simulink model "part2_MAIN_2019_for_ayon_because_he_cant_update_his_matlab"  (R2019a)
settings: Solver=FixedStepAuto  StartTime=0.0  StopTime=300  FixedStep=0.1  RelTol=1e-3
values from neighbouring files (symbols this model uses):
  Af = diag(ti)    [init.m]    (also in init_old.m)
  Aw = [zeros(3) eye(3) ... (first row only)    [get_observer_parameters.m]
  B = [thr1 thr2_x thr2_y thr3 thr4_x thr4_y thr5_x thr5_y]    [B_redistributed.m]    (also in check_alg.m = [1 2 3 4 5 6 7 8; get_observer_parameters.m = [zeros(6,3);zeros(3,3);zeros(3,3);inv(M)])
  change_position_time = 1200    [init.m]    (also in init_old.m)
  Cw = [zeros(3) eye(3)]    [get_observer_parameters.m]
  D = Damping    [init.m]    (also in init_old.m)
  Damping = diag([2.6486e5, 8.8164e5, 3.3774e8])    [init.m]    (also in init_old.m)
  direction_limit = pi/36    (= 0.0872664625997)    [init.m]    (also in init_old.m)
  direction_time_constant = 100    [init.m]    (also in init_old.m)
  dt = 0.1    [get_observer_parameters.m]
  E = [Ew, zeros(6,3) ... (first row only)    [get_observer_parameters.m]
  Gamma = diag(omega_is)    [init.m]    (also in init_old.m)
  gust_limit = 40    [init.m]    (also in init_old.m)
  H = [Cw, eye(3), zeros(3,3) zeros(3,3)]    [get_observer_parameters.m]    (also in quadprog.m = 2*diag([w.' w.' q.' q.' w_alpha.' w_alpha.']); quadprog_basic.m = 2*diag([w.' w.' q.' q.']); quadprog_false.m = 2*diag([w.' w.' q.' q.' w_alpha.' w_alpha.']))
  height = 3    [init.m]    (also in init_old.m)
  inv_M = inv(M)    [get_observer_parameters.m]
  inv_Tb = inv(Tb)    [get_observer_parameters.m]
  kappa = 0.003    [init.m]    (also in init_old.m)
  kappa2 = 0.0026    [init.m]    (also in init_old.m)
  Kd = [1660451.40544401; 3920391.80535684; 1605063439.04156]    [init.m]    (also in init_old.m)
  Ki = [137.081306245593; 3163.274947400198; 335358.448218978]    [init.m]    (also in init_old.m)
  Kp = [75459.3345349083; 277551.73586971; 120744473.878042]    [init.m]    (also in init_old.m)
  L = 1800    [init.m]    (also in init_old.m)
  M = Mass    [init.m]    (also in init_old.m)
  mean_wind_direction = pi    (= 3.14159265359)    [init.m]    (also in init_old.m)
  observer_type = 0    [init.m]    (also in init_old.m)
  Omega = diag([omega_n, omega_n, omega_n])    [get_observer_parameters.m]    (also in init.m = diag(2*omega_is.*zeta_is); init_old.m = diag(2*omega_is.*zeta_is))
  Q = diag([0.1,0.1,pi/180,1e6,1e6,1e9])*10e3    [get_observer_parameters.m]
  R = diag([1,0.1,0.1*pi/180])*10e-3    [get_observer_parameters.m]
  simulation = 7    [init.m]    (also in init_old.m = 1)
  slow_varying_limit = 1    [init.m]    (also in init_old.m)
  slow_varying_time_constant = 100    [init.m]    (also in init_old.m)
  TAU = dt*E    [get_observer_parameters.m]
  Tb = 0.1 * eye(3)    [get_observer_parameters.m]
  thruster_type = 0    [init.m]    (also in init_old.m)
  u10 = 12    [init.m]    (also in init_old.m)
  vessel =     [test.mat]
  wind = 1    [init.m]    (also in init_old.m)
undefined symbols (not defined in the file or in its folder): Hoerner, ModelParams, npf, Param, thrusters, WaveModel
libraries: simulink x49, dspsigops x39, marine_hydro x14, marine_gnc x7
(part 5 of 9)

== system part2_MAIN_2019_for_ayon_because_he_cant_update_his_matlab/ Original/Wind/V_w1 ==
  " " : Constant  Value=mean_wind_direction
  Band-Limited White Noise : simulink/Sources/Band-Limited White Noise  Cov=np_slow_varying  Ts=0.1  seed=[23341]
  Band-Limited White Noise1 : simulink/Sources/Band-Limited White Noise  Cov=np_direction  Ts=0.1  seed=[23341]
  Constant : Constant  Value=u10
  Constant1 : Constant  Value=kappa
  Constant2 : Constant  Value=height
  Constant3 : Constant  Value=u10
  Constant8 : Constant  Value=L
  Constant9 : Constant  Value=kappa2
  Gain : Gain  Gain=1/slow_varying_time_constant
  Gain1 : Gain  Gain=1/direction_time_constant
  Gust : MATLAB Function  TreatAsAtomicUnit=on
  Integrator : Integrator  LimitOutput=on  UpperSaturationLimit=slow_varying_limit  LowerSaturationLimit=-slow_varying_limit
  Integrator1 : Integrator  LimitOutput=on  UpperSaturationLimit=direction_limit  LowerSaturationLimit=-direction_limit
  Mean wind component : MATLAB Function  TreatAsAtomicUnit=on
  Saturation : Saturate  UpperLimit=gust_limit  LowerLimit=-10
  Scope{,1..3} (4 alike) : Scope
  Sum : Sum  Inputs=+|+|+
  Sum1 : Sum  Inputs=|+-
  Sum2 : Sum  Inputs=|+-
  Sum3 : Sum  Inputs=|++
  time : Clock
  wind : Outport
  direction : Outport  Port=2
  wires:
  Constant3/1 -> Mean wind component/1(u10)
  Constant1/1 -> Mean wind component/2(kappa)
  Constant2/1 -> Mean wind component/3(height)
  Mean wind component/1(mean_wind) -> Scope2/1, Sum/2
  Sum/1 -> wind/1
  Integrator/1 -> Scope1/1, Sum/1, Sum1/2
  Band-Limited White Noise/1 -> Sum1/1
  Integrator1/1 -> Sum2/2, Sum3/1
  Band-Limited White Noise1/1 -> Sum2/1
  " "/1 -> Sum3/2
  Sum3/1 -> Scope3/1, direction/1
  Gain1/1 -> Integrator1/1
  Sum2/1 -> Gain1/1
  Gain/1 -> Integrator/1
  Sum1/1 -> Gain/1
  Constant8/1 -> Gust/3(L)
  Gust/1(gust) -> Saturation/1
  Saturation/1 -> Sum/3, Scope/1
  Constant9/1 -> Gust/4(kappa2)
  Constant/1 -> Gust/2(u10)
  time/1 -> Gust/1(time)

== system part2_MAIN_2019_for_ayon_because_he_cant_update_his_matlab/Simulation 1/Current (North - East)/Subsystem ==
  Mux1 : Mux  Inputs=3
  Scope : Scope
  Step1 : Step  Time=0  After=0  SampleTime=0
  Step2 : Step  Time=0  After=-0.2  SampleTime=0
  Step3 : Step  Time=0  After=0  SampleTime=0
  Out1 : Outport
  wires:
  Mux1/1 -> Scope/1, Out1/1
  Step1/1 -> Mux1/1
  Step2/1 -> Mux1/2
  Step3/1 -> Mux1/3

== system part2_MAIN_2019_for_ayon_because_he_cant_update_his_matlab/Simulation 1/Current (North - East)/Subsystem1 ==
  Add : Sum  Inputs=+++
  Cos : Trigonometry  Operator=cos
  Gain : Gain  Gain=pi/180
  Matrix Multiply : Product
  Matrix Multiply1 : Product
  Mux : Mux  Inputs=3
  Ramp : simulink/Sources/Ramp  slope=0.45  start=2  InitialOutput=0
  Ramp1 : simulink/Sources/Ramp  slope=-0.45  start=202  InitialOutput=0
  Scope : Scope  NumInputPorts=3
  Sin : Trigonometry
  Step : Step  Time=2  After=0.5  SampleTime=0
  Step1 : Step  Time=2  Before=180  After=180  SampleTime=0
  Step2 : Step  Time=0  After=0  SampleTime=0
  Out1 : Outport
  wires:
  Step1/1 -> Add/1
  Ramp/1 -> Add/2
  Ramp1/1 -> Add/3
  Step/1 -> Matrix Multiply1/1, Matrix Multiply/1
  Sin/1 -> Matrix Multiply1/2, Scope/1
  Cos/1 -> Matrix Multiply/2, Scope/2
  Matrix Multiply/1 -> Mux/1
  Matrix Multiply1/1 -> Mux/2
  Step2/1 -> Mux/3
  Mux/1 -> Scope/3, Out1/1
  Add/1 -> Gain/1
  Gain/1 -> Sin/1, Cos/1

== system part2_MAIN_2019_for_ayon_because_he_cant_update_his_matlab/Simulation 1/Current (North - East)/Subsystem2 ==
  Mux : Mux  Inputs=3
  Step : Step  Time=0  After=0  SampleTime=0
  Out1 : Outport
  wires:
  Mux/1 -> Out1/1
  Step/1 -> Mux/3, Mux/2, Mux/1

== system part2_MAIN_2019_for_ayon_because_he_cant_update_his_matlab/Simulation 1/Observer/EKF ==
  note: selector
  y : Inport
  U : Inport  Port=2
  Constant : Constant  Value=M
  Constant1 : Constant  Value=D
  Constant10 : Constant  Value=Q
  Constant11 : Constant  Value=dt
  Constant12 : Constant  Value=inv_Tb
  Constant13 : Constant  Value=TAU
  Constant2 : Constant  Value=inv_M
  Constant3 : Constant  Value=Tb
  Constant4 : Constant  Value=Aw
  Constant5 : Constant  Value=Cw
  Constant6 : Constant  Value=B
  Constant7 : Constant  Value=H
  Constant8 : Constant  Value=E
  Constant9 : Constant  Value=R
  MATLAB Function : MATLAB Function  TreatAsAtomicUnit=on
  MATLAB Function1 : MATLAB Function  TreatAsAtomicUnit=on
  Memory : Memory  InitialCondition=zeros(15,1)
  Memory1 : Memory  InitialCondition=eye(15,15)
  Scope : Scope
  Scope2 : Scope
  Subsystem : Subsystem  Commented=on
  Subsystem1 : Subsystem  Commented=on
  Terminator : Terminator
  eta_hat : Outport
  nu_hat : Outport  Port=2
  wires:
  U/1 -> MATLAB Function/2(U)
  MATLAB Function1/1(eta_hat) -> eta_hat/1
  MATLAB Function/3(states_hat) -> MATLAB Function1/1(states_vector)
  MATLAB Function/4(error) -> Scope2/1
  y/1 -> MATLAB Function/1(y)
  MATLAB Function1/2(nu_hat) -> nu_hat/1
  MATLAB Function/2(states_update) -> Memory/1
  Constant/1 -> MATLAB Function/5(M)
  Constant1/1 -> MATLAB Function/6(D)
  Constant2/1 -> MATLAB Function/7(inv_M)
  Constant4/1 -> MATLAB Function/8(Aw)
  Constant3/1 -> MATLAB Function/9(Tb)
  Constant5/1 -> MATLAB Function/10(Cw)
  Constant8/1 -> MATLAB Function/11(E)
  Constant6/1 -> MATLAB Function/12(B)
  Constant7/1 -> MATLAB Function/13(H)
  Constant9/1 -> MATLAB Function/14(R)
  Constant10/1 -> MATLAB Function/15(Q)
  Constant11/1 -> MATLAB Function/16(dt)
  Constant12/1 -> MATLAB Function/17(inv_Tb)
  Constant13/1 -> MATLAB Function/18(TAU)
  Memory/1 -> MATLAB Function/4(states)
  MATLAB Function/1(P_update) -> Memory1/1, Scope/1
  Memory1/1 -> MATLAB Function/3(P)
  MATLAB Function/5(K) -> Terminator/1

== system part2_MAIN_2019_for_ayon_because_he_cant_update_his_matlab/Simulation 1/Observer/Passive Non-Linear ==
  note: eta_observer
  note: nu_observer
  note: Bias Estimator
  note: Wave Estimator: 1st order wave-induced motion
  y : Inport
  tau_est : Inport  Port=2
  Add : Sum
  Add1 : Sum  Inputs=++-
  Aw : Gain  Gain=WaveModel.A_w  Multiplication=Matrix(K*u)
  Cw : Gain  Gain=WaveModel.C_w  Multiplication=Matrix(K*u)
  Damping : Gain  Gain=Damping  Multiplication=Matrix(K*u)
  Integrator{,1..3} (4 alike) : Integrator
  K1 : Gain  Gain=npf.K_1  Multiplication=Matrix(K*u)
  K2 : Gain  Gain=npf.K_2  Multiplication=Matrix(K*u)
  K3 : Gain  Gain=npf.K_3  Multiplication=Matrix(K*u)
  K4 : Gain  Gain=npf.K_4  Multiplication=Matrix(K*u)
  M_inv : Gain  Gain=inv(ModelParams.Mass)  Multiplication=Matrix(K*u)
  Matrix Multiply : Product  Multiplication=Matrix(*)
  Matrix Multiply1 : Product  Multiplication=Matrix(*)
  Matrix Multiply2 : Product  Multiplication=Matrix(*)
  R_psi : MATLAB Function  TreatAsAtomicUnit=on
  R_psi_T : MATLAB Function  TreatAsAtomicUnit=on
  Subsystem : Subsystem
  Sum : Sum  Inputs=|++
  Sum1 : Sum  Inputs=|+-
  Sum2 : Sum  Inputs=|++
  Sum3 : Sum  Inputs=|++
  Sum4 : Sum  Inputs=|+-
  inv(Tb) : Gain  Gain=inv(Param.Tb)  Multiplication=Matrix(K*u)
  eta_hat : Outport
  nu_hat : Outport  Port=2
  wires:
  Matrix Multiply/1 -> Sum/1
  Matrix Multiply1/1 -> Add/2
  Matrix Multiply2/1 -> Add1/1  "R'b_hat"
  R_psi_T/1(y) -> Matrix Multiply/1, Matrix Multiply2/2
  Add1/1 -> M_inv/1
  Damping/1 -> Add1/3
  R_psi/1(y) -> Matrix Multiply1/1
  Sum/1 -> Add1/2  "R'k4y + tau"
  Add/1 -> Integrator3/1  "eta_hat_dot"
  inv(Tb)/1 -> Sum1/2
  y/1 -> Subsystem/1(y), Sum4/1  "y"
  Aw/1 -> Sum2/2
  K3/1 -> Sum1/1
  Cw/1 -> Sum3/1
  Integrator1/1 -> Cw/1, Aw/1  "zeta_hat"
  Sum1/1 -> Integrator2/1  "b_hat_dot"
  Integrator/1 -> nu_hat/1, Damping/1, Matrix Multiply1/2  "nu_hat"
  Sum4/1 -> K1/1, K2/1, K3/1, K4/1  "y_obs"
  Sum3/1 -> Sum4/2  "y_hat"
  Integrator3/1 -> eta_hat/1, Sum3/2  "eta_hat"
  Sum2/1 -> Integrator1/1
  K2/1 -> Add/1
  K4/1 -> Matrix Multiply/2
  M_inv/1 -> Integrator/1  "nu_hat_dot"
  Integrator2/1 -> inv(Tb)/1, Matrix Multiply2/1  "b_hat"
  tau_est/1 -> Sum/2
  K1/1 -> Sum2/1
  Subsystem/1(Out1) -> R_psi/1(u), R_psi_T/1(u)

== system part2_MAIN_2019_for_ayon_because_he_cant_update_his_matlab/Simulation 1/Observer/Subsystem ==
  In1 : Inport
  Demux : Demux  Outputs=6
  Mux : Mux  Inputs=3
  Terminator : Terminator
  Terminator1 : Terminator
  Terminator2 : Terminator
  Out1 : Outport
  wires:
  Mux/1 -> Out1/1
  Demux/6 -> Mux/3
  Demux/5 -> Terminator2/1
  Demux/2 -> Mux/2
  Demux/1 -> Mux/1
  Demux/3 -> Terminator/1
  In1/1 -> Demux/1
  Demux/4 -> Terminator1/1

== system part2_MAIN_2019_for_ayon_because_he_cant_update_his_matlab/Simulation 1/Reference Model/Simulation Selector ==
  Simulation 4 : Subsystem
  Out1 : Outport
  wires:
  Simulation 4/1(Out1) -> Out1/1

== system part2_MAIN_2019_for_ayon_because_he_cant_update_his_matlab/Simulation 1/Thrust Allocation/Unwrap ==
  alpha : Inport
  Demux : Demux  Outputs=5
  Mux : Mux  Inputs=5
  Unwrap : dspsigops/Unwrap  tol=pi  InputProcessing=Columns as channels (frame based)  running=off
  Unwrap1 : dspsigops/Unwrap  tol=pi  InputProcessing=Columns as channels (frame based)  running=off
  Unwrap2 : dspsigops/Unwrap  tol=pi  InputProcessing=Columns as channels (frame based)  running=off
  alpha [rad] : Outport
  wires:
  alpha/1 -> Demux/1
  Mux/1 -> alpha [rad]/1
  Demux/1 -> Mux/1
  Demux/4 -> Unwrap2/1
  Unwrap2/1 -> Mux/4
  Demux/5 -> Unwrap/1
  Unwrap/1 -> Mux/5
  Demux/3 -> Mux/3
  Demux/2 -> Unwrap1/1
  Unwrap1/1 -> Mux/2

== system part2_MAIN_2019_for_ayon_because_he_cant_update_his_matlab/Simulation 1/Thrust Allocation/Unwrap1 ==
  alpha : Inport
  Demux : Demux  Outputs=5
  Mux : Mux  Inputs=5
  Unwrap : dspsigops/Unwrap  tol=pi  InputProcessing=Columns as channels (frame based)  running=off
  Unwrap1 : dspsigops/Unwrap  tol=pi  InputProcessing=Columns as channels (frame based)  running=off
  Unwrap2 : dspsigops/Unwrap  tol=pi  InputProcessing=Columns as channels (frame based)  running=off
  alpha [rad] : Outport
  wires:
  Unwrap1/1 -> Mux/2
  Demux/2 -> Unwrap1/1
  Demux/3 -> Mux/3
  Unwrap/1 -> Mux/5
  Demux/5 -> Unwrap/1
  Unwrap2/1 -> Mux/4
  Demux/4 -> Unwrap2/1
  Demux/1 -> Mux/1
  Mux/1 -> alpha [rad]/1
  alpha/1 -> Demux/1

== system part2_MAIN_2019_for_ayon_because_he_cant_update_his_matlab/Simulation 1/Wind/V_w1 ==
  " " : Constant  Value=mean_wind_direction
  Band-Limited White Noise : simulink/Sources/Band-Limited White Noise  Cov=np_slow_varying  Ts=0.1  seed=[23341]
  Band-Limited White Noise1 : simulink/Sources/Band-Limited White Noise  Cov=np_direction  Ts=0.1  seed=[23341]
  Constant : Constant  Value=u10
  Constant1 : Constant  Value=kappa
  Constant2 : Constant  Value=height
  Constant3 : Constant  Value=u10
  Constant8 : Constant  Value=L
  Constant9 : Constant  Value=kappa2
  Gain : Gain  Gain=1/slow_varying_time_constant
  Gain1 : Gain  Gain=1/direction_time_constant
  Gust : MATLAB Function  TreatAsAtomicUnit=on
  Integrator : Integrator  LimitOutput=on  UpperSaturationLimit=slow_varying_limit  LowerSaturationLimit=-slow_varying_limit
  Integrator1 : Integrator  LimitOutput=on  UpperSaturationLimit=direction_limit  LowerSaturationLimit=-direction_limit
  Mean wind component : MATLAB Function  TreatAsAtomicUnit=on
  Saturation : Saturate  UpperLimit=gust_limit  LowerLimit=-10
  Scope{,1..3} (4 alike) : Scope
  Sum : Sum  Inputs=+|+|+
  Sum1 : Sum  Inputs=|+-
  Sum2 : Sum  Inputs=|+-
  Sum3 : Sum  Inputs=|++
  time : Clock
  wind : Outport
  direction : Outport  Port=2
  wires:
  Constant3/1 -> Mean wind component/1(u10)
  Constant1/1 -> Mean wind component/2(kappa)
  Constant2/1 -> Mean wind component/3(height)
  Mean wind component/1(mean_wind) -> Scope2/1, Sum/2
  Sum/1 -> wind/1
  Integrator/1 -> Scope1/1, Sum/1, Sum1/2
  Band-Limited White Noise/1 -> Sum1/1
  Integrator1/1 -> Sum2/2, Sum3/1
  Band-Limited White Noise1/1 -> Sum2/1
  " "/1 -> Sum3/2
  Sum3/1 -> Scope3/1, direction/1
  Gain1/1 -> Integrator1/1
  Sum2/1 -> Gain1/1
  Gain/1 -> Integrator/1
  Sum1/1 -> Gain/1
  Constant8/1 -> Gust/3(L)
  Gust/1(gust) -> Saturation/1
  Saturation/1 -> Sum/3, Scope/1
  Constant9/1 -> Gust/4(kappa2)
  Constant/1 -> Gust/2(u10)
  time/1 -> Gust/1(time)

== system part2_MAIN_2019_for_ayon_because_he_cant_update_his_matlab/Simulation 2/Current (North - East)/Subsystem ==
  Mux1 : Mux  Inputs=3
  Scope : Scope
  Step1 : Step  Time=0  After=0  SampleTime=0
  Step2 : Step  Time=0  After=-0.2  SampleTime=0
  Step3 : Step  Time=0  After=0  SampleTime=0
  Out1 : Outport
  wires:
  Mux1/1 -> Scope/1, Out1/1
  Step1/1 -> Mux1/1
  Step2/1 -> Mux1/2
  Step3/1 -> Mux1/3

== system part2_MAIN_2019_for_ayon_because_he_cant_update_his_matlab/Simulation 2/Current (North - East)/Subsystem1 ==
  Add : Sum  Inputs=+++
  Cos : Trigonometry  Operator=cos
  Gain : Gain  Gain=pi/180
  Matrix Multiply : Product
  Matrix Multiply1 : Product
  Mux : Mux  Inputs=3
  Ramp : simulink/Sources/Ramp  slope=0.45  start=2  InitialOutput=0
  Ramp1 : simulink/Sources/Ramp  slope=-0.45  start=202  InitialOutput=0
  Scope : Scope  NumInputPorts=3
  Sin : Trigonometry
  Step : Step  Time=2  After=0.5  SampleTime=0
  Step1 : Step  Time=2  Before=180  After=180  SampleTime=0
  Step2 : Step  Time=0  After=0  SampleTime=0
  Out1 : Outport
  wires:
  Step1/1 -> Add/1
  Ramp/1 -> Add/2
  Ramp1/1 -> Add/3
  Step/1 -> Matrix Multiply1/1, Matrix Multiply/1
  Sin/1 -> Matrix Multiply1/2, Scope/1
  Cos/1 -> Matrix Multiply/2, Scope/2
  Matrix Multiply/1 -> Mux/1
  Matrix Multiply1/1 -> Mux/2
  Step2/1 -> Mux/3
  Mux/1 -> Scope/3, Out1/1
  Add/1 -> Gain/1
  Gain/1 -> Sin/1, Cos/1

== system part2_MAIN_2019_for_ayon_because_he_cant_update_his_matlab/Simulation 2/Current (North - East)/Subsystem2 ==
  Mux : Mux  Inputs=3
  Step : Step  Time=0  After=0  SampleTime=0
  Out1 : Outport
  wires:
  Mux/1 -> Out1/1
  Step/1 -> Mux/3, Mux/2, Mux/1

== system part2_MAIN_2019_for_ayon_because_he_cant_update_his_matlab/Simulation 2/Observer/EKF ==
  note: selector
  y : Inport
  U : Inport  Port=2
  Constant : Constant  Value=M
  Constant1 : Constant  Value=D
  Constant10 : Constant  Value=Q
  Constant11 : Constant  Value=dt
  Constant12 : Constant  Value=inv_Tb
  Constant13 : Constant  Value=TAU
  Constant2 : Constant  Value=inv_M
  Constant3 : Constant  Value=Tb
  Constant4 : Constant  Value=Aw
  Constant5 : Constant  Value=Cw
  Constant6 : Constant  Value=B
  Constant7 : Constant  Value=H
  Constant8 : Constant  Value=E
  Constant9 : Constant  Value=R
  MATLAB Function : MATLAB Function  TreatAsAtomicUnit=on
  MATLAB Function1 : MATLAB Function  TreatAsAtomicUnit=on
  Memory : Memory  InitialCondition=zeros(15,1)
  Memory1 : Memory  InitialCondition=eye(15,15)
  Scope : Scope
  Scope2 : Scope
  Subsystem : Subsystem  Commented=on
  Subsystem1 : Subsystem  Commented=on
  Terminator : Terminator
  eta_hat : Outport
  nu_hat : Outport  Port=2
  wires:
  U/1 -> MATLAB Function/2(U)
  MATLAB Function1/1(eta_hat) -> eta_hat/1
  MATLAB Function/3(states_hat) -> MATLAB Function1/1(states_vector)
  MATLAB Function/4(error) -> Scope2/1
  y/1 -> MATLAB Function/1(y)
  MATLAB Function1/2(nu_hat) -> nu_hat/1
  MATLAB Function/2(states_update) -> Memory/1
  Constant/1 -> MATLAB Function/5(M)
  Constant1/1 -> MATLAB Function/6(D)
  Constant2/1 -> MATLAB Function/7(inv_M)
  Constant4/1 -> MATLAB Function/8(Aw)
  Constant3/1 -> MATLAB Function/9(Tb)
  Constant5/1 -> MATLAB Function/10(Cw)
  Constant8/1 -> MATLAB Function/11(E)
  Constant6/1 -> MATLAB Function/12(B)
  Constant7/1 -> MATLAB Function/13(H)
  Constant9/1 -> MATLAB Function/14(R)
  Constant10/1 -> MATLAB Function/15(Q)
  Constant11/1 -> MATLAB Function/16(dt)
  Constant12/1 -> MATLAB Function/17(inv_Tb)
  Constant13/1 -> MATLAB Function/18(TAU)
  Memory/1 -> MATLAB Function/4(states)
  MATLAB Function/1(P_update) -> Memory1/1, Scope/1
  Memory1/1 -> MATLAB Function/3(P)
  MATLAB Function/5(K) -> Terminator/1

== system part2_MAIN_2019_for_ayon_because_he_cant_update_his_matlab/Simulation 2/Observer/Passive Non-Linear ==
  note: eta_observer
  note: nu_observer
  note: Bias Estimator
  note: Wave Estimator: 1st order wave-induced motion
  y : Inport
  tau_est : Inport  Port=2
  Add : Sum
  Add1 : Sum  Inputs=++-
  Aw : Gain  Gain=WaveModel.A_w  Multiplication=Matrix(K*u)
  Cw : Gain  Gain=WaveModel.C_w  Multiplication=Matrix(K*u)
  Damping : Gain  Gain=Damping  Multiplication=Matrix(K*u)
  Integrator{,1..3} (4 alike) : Integrator
  K1 : Gain  Gain=npf.K_1  Multiplication=Matrix(K*u)
  K2 : Gain  Gain=npf.K_2  Multiplication=Matrix(K*u)
  K3 : Gain  Gain=npf.K_3  Multiplication=Matrix(K*u)
  K4 : Gain  Gain=npf.K_4  Multiplication=Matrix(K*u)
  M_inv : Gain  Gain=inv(ModelParams.Mass)  Multiplication=Matrix(K*u)
  Matrix Multiply : Product  Multiplication=Matrix(*)
  Matrix Multiply1 : Product  Multiplication=Matrix(*)
  Matrix Multiply2 : Product  Multiplication=Matrix(*)
  R_psi : MATLAB Function  TreatAsAtomicUnit=on
  R_psi_T : MATLAB Function  TreatAsAtomicUnit=on
  Subsystem : Subsystem
  Sum : Sum  Inputs=|++
  Sum1 : Sum  Inputs=|+-
  Sum2 : Sum  Inputs=|++
  Sum3 : Sum  Inputs=|++
  Sum4 : Sum  Inputs=|+-
  inv(Tb) : Gain  Gain=inv(Param.Tb)  Multiplication=Matrix(K*u)
  eta_hat : Outport
  nu_hat : Outport  Port=2
  wires:
  Matrix Multiply/1 -> Sum/1
  Matrix Multiply1/1 -> Add/2
  Matrix Multiply2/1 -> Add1/1  "R'b_hat"
  R_psi_T/1(y) -> Matrix Multiply/1, Matrix Multiply2/2
  Add1/1 -> M_inv/1
  Damping/1 -> Add1/3
  R_psi/1(y) -> Matrix Multiply1/1
  Sum/1 -> Add1/2  "R'k4y + tau"
  Add/1 -> Integrator3/1  "eta_hat_dot"
  inv(Tb)/1 -> Sum1/2
  y/1 -> Subsystem/1(y), Sum4/1  "y"
  Aw/1 -> Sum2/2
  K3/1 -> Sum1/1
  Cw/1 -> Sum3/1
  Integrator1/1 -> Cw/1, Aw/1  "zeta_hat"
  Sum1/1 -> Integrator2/1  "b_hat_dot"
  Integrator/1 -> nu_hat/1, Damping/1, Matrix Multiply1/2  "nu_hat"
  Sum4/1 -> K1/1, K2/1, K3/1, K4/1  "y_obs"
  Sum3/1 -> Sum4/2  "y_hat"
  Integrator3/1 -> eta_hat/1, Sum3/2  "eta_hat"
  Sum2/1 -> Integrator1/1
  K2/1 -> Add/1
  K4/1 -> Matrix Multiply/2
  M_inv/1 -> Integrator/1  "nu_hat_dot"
  Integrator2/1 -> inv(Tb)/1, Matrix Multiply2/1  "b_hat"
  tau_est/1 -> Sum/2
  K1/1 -> Sum2/1
  Subsystem/1(Out1) -> R_psi/1(u), R_psi_T/1(u)

== system part2_MAIN_2019_for_ayon_because_he_cant_update_his_matlab/Simulation 2/Observer/Subsystem ==
  In1 : Inport
  Demux : Demux  Outputs=6
  Mux : Mux  Inputs=3
  Terminator : Terminator
  Terminator1 : Terminator
  Terminator2 : Terminator
  Out1 : Outport
  wires:
  Mux/1 -> Out1/1
  Demux/6 -> Mux/3
  Demux/5 -> Terminator2/1
  Demux/2 -> Mux/2
  Demux/1 -> Mux/1
  Demux/3 -> Terminator/1
  In1/1 -> Demux/1
  Demux/4 -> Terminator1/1

== system part2_MAIN_2019_for_ayon_because_he_cant_update_his_matlab/Simulation 2/Reference Model/Simulation Selector ==
  Simulation 4 : Subsystem
  Out1 : Outport
  wires:
  Simulation 4/1(Out1) -> Out1/1

== system part2_MAIN_2019_for_ayon_because_he_cant_update_his_matlab/Simulation 2/Thrust Allocation/Unwrap ==
  alpha : Inport
  Demux : Demux  Outputs=5
  Mux : Mux  Inputs=5
  Unwrap : dspsigops/Unwrap  tol=pi  InputProcessing=Columns as channels (frame based)  running=off
  Unwrap1 : dspsigops/Unwrap  tol=pi  InputProcessing=Columns as channels (frame based)  running=off
  Unwrap2 : dspsigops/Unwrap  tol=pi  InputProcessing=Columns as channels (frame based)  running=off
  alpha [rad] : Outport
  wires:
  alpha/1 -> Demux/1
  Mux/1 -> alpha [rad]/1
  Demux/1 -> Mux/1
  Demux/4 -> Unwrap2/1
  Unwrap2/1 -> Mux/4
  Demux/5 -> Unwrap/1
  Unwrap/1 -> Mux/5
  Demux/3 -> Mux/3
  Demux/2 -> Unwrap1/1
  Unwrap1/1 -> Mux/2

== system part2_MAIN_2019_for_ayon_because_he_cant_update_his_matlab/Simulation 2/Thrust Allocation/Unwrap1 ==
  alpha : Inport
  Demux : Demux  Outputs=5
  Mux : Mux  Inputs=5
  Unwrap : dspsigops/Unwrap  tol=pi  InputProcessing=Columns as channels (frame based)  running=off
  Unwrap1 : dspsigops/Unwrap  tol=pi  InputProcessing=Columns as channels (frame based)  running=off
  Unwrap2 : dspsigops/Unwrap  tol=pi  InputProcessing=Columns as channels (frame based)  running=off
  alpha [rad] : Outport
  wires:
  Unwrap1/1 -> Mux/2
  Demux/2 -> Unwrap1/1
  Demux/3 -> Mux/3
  Unwrap/1 -> Mux/5
  Demux/5 -> Unwrap/1
  Unwrap2/1 -> Mux/4
  Demux/4 -> Unwrap2/1
  Demux/1 -> Mux/1
  Mux/1 -> alpha [rad]/1
  alpha/1 -> Demux/1

== system part2_MAIN_2019_for_ayon_because_he_cant_update_his_matlab/Simulation 2/Wind/V_w1 ==
  " " : Constant  Value=mean_wind_direction
  Band-Limited White Noise : simulink/Sources/Band-Limited White Noise  Cov=np_slow_varying  Ts=0.1  seed=[23341]
  Band-Limited White Noise1 : simulink/Sources/Band-Limited White Noise  Cov=np_direction  Ts=0.1  seed=[23341]
  Constant : Constant  Value=u10
  Constant1 : Constant  Value=kappa
  Constant2 : Constant  Value=height
  Constant3 : Constant  Value=u10
  Constant8 : Constant  Value=L
  Constant9 : Constant  Value=kappa2
  Gain : Gain  Gain=1/slow_varying_time_constant
  Gain1 : Gain  Gain=1/direction_time_constant
  Gust : MATLAB Function  TreatAsAtomicUnit=on
  Integrator : Integrator  LimitOutput=on  UpperSaturationLimit=slow_varying_limit  LowerSaturationLimit=-slow_varying_limit
  Integrator1 : Integrator  LimitOutput=on  UpperSaturationLimit=direction_limit  LowerSaturationLimit=-direction_limit
  Mean wind component : MATLAB Function  TreatAsAtomicUnit=on
  Saturation : Saturate  UpperLimit=gust_limit  LowerLimit=-10
  Scope{,1..3} (4 alike) : Scope
  Sum : Sum  Inputs=+|+|+
  Sum1 : Sum  Inputs=|+-
  Sum2 : Sum  Inputs=|+-
  Sum3 : Sum  Inputs=|++
  time : Clock
  wind : Outport
  direction : Outport  Port=2
  wires:
  Constant3/1 -> Mean wind component/1(u10)
  Constant1/1 -> Mean wind component/2(kappa)
  Constant2/1 -> Mean wind component/3(height)
  Mean wind component/1(mean_wind) -> Scope2/1, Sum/2
  Sum/1 -> wind/1
  Integrator/1 -> Scope1/1, Sum/1, Sum1/2
  Band-Limited White Noise/1 -> Sum1/1
  Integrator1/1 -> Sum2/2, Sum3/1
  Band-Limited White Noise1/1 -> Sum2/1
  " "/1 -> Sum3/2
  Sum3/1 -> Scope3/1, direction/1
  Gain1/1 -> Integrator1/1
  Sum2/1 -> Gain1/1
  Gain/1 -> Integrator/1
  Sum1/1 -> Gain/1
  Constant8/1 -> Gust/3(L)
  Gust/1(gust) -> Saturation/1
  Saturation/1 -> Sum/3, Scope/1
  Constant9/1 -> Gust/4(kappa2)
  Constant/1 -> Gust/2(u10)
  time/1 -> Gust/1(time)

== system part2_MAIN_2019_for_ayon_because_he_cant_update_his_matlab/Simulation 3/Current (North - East)/Subsystem ==
  Mux1 : Mux  Inputs=3
  Scope : Scope
  Step1 : Step  Time=0  After=0  SampleTime=0
  Step2 : Step  Time=0  After=-0.2  SampleTime=0
  Step3 : Step  Time=0  After=0  SampleTime=0
  Out1 : Outport
  wires:
  Mux1/1 -> Scope/1, Out1/1
  Step1/1 -> Mux1/1
  Step2/1 -> Mux1/2
  Step3/1 -> Mux1/3

== system part2_MAIN_2019_for_ayon_because_he_cant_update_his_matlab/Simulation 3/Current (North - East)/Subsystem1 ==
  Add : Sum  Inputs=+++
  Cos : Trigonometry  Operator=cos
  Gain : Gain  Gain=pi/180
  Matrix Multiply : Product
  Matrix Multiply1 : Product
  Mux : Mux  Inputs=3
  Ramp : simulink/Sources/Ramp  slope=0.45  start=2  InitialOutput=0
  Ramp1 : simulink/Sources/Ramp  slope=-0.45  start=202  InitialOutput=0
  Scope : Scope  NumInputPorts=3
  Sin : Trigonometry
  Step : Step  Time=2  After=0.5  SampleTime=0
  Step1 : Step  Time=2  Before=180  After=180  SampleTime=0
  Step2 : Step  Time=0  After=0  SampleTime=0
  Out1 : Outport
  wires:
  Step1/1 -> Add/1
  Ramp/1 -> Add/2
  Ramp1/1 -> Add/3
  Step/1 -> Matrix Multiply1/1, Matrix Multiply/1
  Sin/1 -> Matrix Multiply1/2, Scope/1
  Cos/1 -> Matrix Multiply/2, Scope/2
  Matrix Multiply/1 -> Mux/1
  Matrix Multiply1/1 -> Mux/2
  Step2/1 -> Mux/3
  Mux/1 -> Scope/3, Out1/1
  Add/1 -> Gain/1
  Gain/1 -> Sin/1, Cos/1

== system part2_MAIN_2019_for_ayon_because_he_cant_update_his_matlab/Simulation 3/Current (North - East)/Subsystem2 ==
  Mux : Mux  Inputs=3
  Step : Step  Time=0  After=0  SampleTime=0
  Out1 : Outport
  wires:
  Mux/1 -> Out1/1
  Step/1 -> Mux/3, Mux/2, Mux/1

== system part2_MAIN_2019_for_ayon_because_he_cant_update_his_matlab/Simulation 3/Observer/EKF ==
  note: selector
  y : Inport
  U : Inport  Port=2
  Constant : Constant  Value=M
  Constant1 : Constant  Value=D
  Constant10 : Constant  Value=Q
  Constant11 : Constant  Value=dt
  Constant12 : Constant  Value=inv_Tb
  Constant13 : Constant  Value=TAU
  Constant2 : Constant  Value=inv_M
  Constant3 : Constant  Value=Tb
  Constant4 : Constant  Value=Aw
  Constant5 : Constant  Value=Cw
  Constant6 : Constant  Value=B
  Constant7 : Constant  Value=H
  Constant8 : Constant  Value=E
  Constant9 : Constant  Value=R
  MATLAB Function : MATLAB Function  TreatAsAtomicUnit=on
  MATLAB Function1 : MATLAB Function  TreatAsAtomicUnit=on
  Memory : Memory  InitialCondition=zeros(15,1)
  Memory1 : Memory  InitialCondition=eye(15,15)
  Scope : Scope
  Scope2 : Scope
  Subsystem : Subsystem  Commented=on
  Subsystem1 : Subsystem  Commented=on
  Terminator : Terminator
  eta_hat : Outport
  nu_hat : Outport  Port=2
  wires:
  U/1 -> MATLAB Function/2(U)
  MATLAB Function1/1(eta_hat) -> eta_hat/1
  MATLAB Function/3(states_hat) -> MATLAB Function1/1(states_vector)
  MATLAB Function/4(error) -> Scope2/1
  y/1 -> MATLAB Function/1(y)
  MATLAB Function1/2(nu_hat) -> nu_hat/1
  MATLAB Function/2(states_update) -> Memory/1
  Constant/1 -> MATLAB Function/5(M)
  Constant1/1 -> MATLAB Function/6(D)
  Constant2/1 -> MATLAB Function/7(inv_M)
  Constant4/1 -> MATLAB Function/8(Aw)
  Constant3/1 -> MATLAB Function/9(Tb)
  Constant5/1 -> MATLAB Function/10(Cw)
  Constant8/1 -> MATLAB Function/11(E)
  Constant6/1 -> MATLAB Function/12(B)
  Constant7/1 -> MATLAB Function/13(H)
  Constant9/1 -> MATLAB Function/14(R)
  Constant10/1 -> MATLAB Function/15(Q)
  Constant11/1 -> MATLAB Function/16(dt)
  Constant12/1 -> MATLAB Function/17(inv_Tb)
  Constant13/1 -> MATLAB Function/18(TAU)
  Memory/1 -> MATLAB Function/4(states)
  MATLAB Function/1(P_update) -> Memory1/1, Scope/1
  Memory1/1 -> MATLAB Function/3(P)
  MATLAB Function/5(K) -> Terminator/1

== system part2_MAIN_2019_for_ayon_because_he_cant_update_his_matlab/Simulation 3/Observer/Passive Non-Linear ==
  note: eta_observer
  note: nu_observer
  note: Bias Estimator
  note: Wave Estimator: 1st order wave-induced motion
  y : Inport
  tau_est : Inport  Port=2
  Add : Sum
  Add1 : Sum  Inputs=++-
  Aw : Gain  Gain=WaveModel.A_w  Multiplication=Matrix(K*u)
  Cw : Gain  Gain=WaveModel.C_w  Multiplication=Matrix(K*u)
  Damping : Gain  Gain=Damping  Multiplication=Matrix(K*u)
  Integrator{,1..3} (4 alike) : Integrator
  K1 : Gain  Gain=npf.K_1  Multiplication=Matrix(K*u)
  K2 : Gain  Gain=npf.K_2  Multiplication=Matrix(K*u)
  K3 : Gain  Gain=npf.K_3  Multiplication=Matrix(K*u)
  K4 : Gain  Gain=npf.K_4  Multiplication=Matrix(K*u)
  M_inv : Gain  Gain=inv(ModelParams.Mass)  Multiplication=Matrix(K*u)
  Matrix Multiply : Product  Multiplication=Matrix(*)
  Matrix Multiply1 : Product  Multiplication=Matrix(*)
  Matrix Multiply2 : Product  Multiplication=Matrix(*)
  R_psi : MATLAB Function  TreatAsAtomicUnit=on
  R_psi_T : MATLAB Function  TreatAsAtomicUnit=on
  Subsystem : Subsystem
  Sum : Sum  Inputs=|++
  Sum1 : Sum  Inputs=|+-
  Sum2 : Sum  Inputs=|++
  Sum3 : Sum  Inputs=|++
  Sum4 : Sum  Inputs=|+-
  inv(Tb) : Gain  Gain=inv(Param.Tb)  Multiplication=Matrix(K*u)
  eta_hat : Outport
  nu_hat : Outport  Port=2
  wires:
  Matrix Multiply/1 -> Sum/1
  Matrix Multiply1/1 -> Add/2
  Matrix Multiply2/1 -> Add1/1  "R'b_hat"
  R_psi_T/1(y) -> Matrix Multiply/1, Matrix Multiply2/2
  Add1/1 -> M_inv/1
  Damping/1 -> Add1/3
  R_psi/1(y) -> Matrix Multiply1/1
  Sum/1 -> Add1/2  "R'k4y + tau"
  Add/1 -> Integrator3/1  "eta_hat_dot"
  inv(Tb)/1 -> Sum1/2
  y/1 -> Subsystem/1(y), Sum4/1  "y"
  Aw/1 -> Sum2/2
  K3/1 -> Sum1/1
  Cw/1 -> Sum3/1
  Integrator1/1 -> Cw/1, Aw/1  "zeta_hat"
  Sum1/1 -> Integrator2/1  "b_hat_dot"
  Integrator/1 -> nu_hat/1, Damping/1, Matrix Multiply1/2  "nu_hat"
  Sum4/1 -> K1/1, K2/1, K3/1, K4/1  "y_obs"
  Sum3/1 -> Sum4/2  "y_hat"
  Integrator3/1 -> eta_hat/1, Sum3/2  "eta_hat"
  Sum2/1 -> Integrator1/1
  K2/1 -> Add/1
  K4/1 -> Matrix Multiply/2
  M_inv/1 -> Integrator/1  "nu_hat_dot"
  Integrator2/1 -> inv(Tb)/1, Matrix Multiply2/1  "b_hat"
  tau_est/1 -> Sum/2
  K1/1 -> Sum2/1
  Subsystem/1(Out1) -> R_psi/1(u), R_psi_T/1(u)

== system part2_MAIN_2019_for_ayon_because_he_cant_update_his_matlab/Simulation 3/Observer/Subsystem ==
  In1 : Inport
  Demux : Demux  Outputs=6
  Mux : Mux  Inputs=3
  Terminator : Terminator
  Terminator1 : Terminator
  Terminator2 : Terminator
  Out1 : Outport
  wires:
  Mux/1 -> Out1/1
  Demux/6 -> Mux/3
  Demux/5 -> Terminator2/1
  Demux/2 -> Mux/2
  Demux/1 -> Mux/1
  Demux/3 -> Terminator/1
  In1/1 -> Demux/1
  Demux/4 -> Terminator1/1

== system part2_MAIN_2019_for_ayon_because_he_cant_update_his_matlab/Simulation 3/Reference Model/Simulation Selector ==
  Simulation 4 : Subsystem
  Out1 : Outport
  wires:
  Simulation 4/1(Out1) -> Out1/1

== system part2_MAIN_2019_for_ayon_because_he_cant_update_his_matlab/Simulation 3/Thrust Allocation/Unwrap ==
  alpha : Inport
  Demux : Demux  Outputs=5
  Mux : Mux  Inputs=5
  Unwrap : dspsigops/Unwrap  tol=pi  InputProcessing=Columns as channels (frame based)  running=off
  Unwrap1 : dspsigops/Unwrap  tol=pi  InputProcessing=Columns as channels (frame based)  running=off
  Unwrap2 : dspsigops/Unwrap  tol=pi  InputProcessing=Columns as channels (frame based)  running=off
  alpha [rad] : Outport
  wires:
  alpha/1 -> Demux/1
  Mux/1 -> alpha [rad]/1
  Demux/1 -> Mux/1
  Demux/4 -> Unwrap2/1
  Unwrap2/1 -> Mux/4
  Demux/5 -> Unwrap/1
  Unwrap/1 -> Mux/5
  Demux/3 -> Mux/3
  Demux/2 -> Unwrap1/1
  Unwrap1/1 -> Mux/2

== system part2_MAIN_2019_for_ayon_because_he_cant_update_his_matlab/Simulation 3/Thrust Allocation/Unwrap1 ==
  alpha : Inport
  Demux : Demux  Outputs=5
  Mux : Mux  Inputs=5
  Unwrap : dspsigops/Unwrap  tol=pi  InputProcessing=Columns as channels (frame based)  running=off
  Unwrap1 : dspsigops/Unwrap  tol=pi  InputProcessing=Columns as channels (frame based)  running=off
  Unwrap2 : dspsigops/Unwrap  tol=pi  InputProcessing=Columns as channels (frame based)  running=off
  alpha [rad] : Outport
  wires:
  Unwrap1/1 -> Mux/2
  Demux/2 -> Unwrap1/1
  Demux/3 -> Mux/3
  Unwrap/1 -> Mux/5
  Demux/5 -> Unwrap/1
  Unwrap2/1 -> Mux/4
  Demux/4 -> Unwrap2/1
  Demux/1 -> Mux/1
  Mux/1 -> alpha [rad]/1
  alpha/1 -> Demux/1

== system part2_MAIN_2019_for_ayon_because_he_cant_update_his_matlab/Simulation 3/Wind/V_w1 ==
  " " : Constant  Value=mean_wind_direction
  Band-Limited White Noise : simulink/Sources/Band-Limited White Noise  Cov=np_slow_varying  Ts=0.1  seed=[23341]
  Band-Limited White Noise1 : simulink/Sources/Band-Limited White Noise  Cov=np_direction  Ts=0.1  seed=[23341]
  Constant : Constant  Value=u10
  Constant1 : Constant  Value=kappa
  Constant2 : Constant  Value=height
  Constant3 : Constant  Value=u10
  Constant8 : Constant  Value=L
  Constant9 : Constant  Value=kappa2
  Gain : Gain  Gain=1/slow_varying_time_constant
  Gain1 : Gain  Gain=1/direction_time_constant
  Gust : MATLAB Function  TreatAsAtomicUnit=on
  Integrator : Integrator  LimitOutput=on  UpperSaturationLimit=slow_varying_limit  LowerSaturationLimit=-slow_varying_limit
  Integrator1 : Integrator  LimitOutput=on  UpperSaturationLimit=direction_limit  LowerSaturationLimit=-direction_limit
  Mean wind component : MATLAB Function  TreatAsAtomicUnit=on
  Saturation : Saturate  UpperLimit=gust_limit  LowerLimit=-10
  Scope{,1..3} (4 alike) : Scope
  Sum : Sum  Inputs=+|+|+
  Sum1 : Sum  Inputs=|+-
  Sum2 : Sum  Inputs=|+-
  Sum3 : Sum  Inputs=|++
  time : Clock
  wind : Outport
  direction : Outport  Port=2
  wires:
  Constant3/1 -> Mean wind component/1(u10)
  Constant1/1 -> Mean wind component/2(kappa)
  Constant2/1 -> Mean wind component/3(height)
  Mean wind component/1(mean_wind) -> Scope2/1, Sum/2
  Sum/1 -> wind/1
  Integrator/1 -> Scope1/1, Sum/1, Sum1/2
  Band-Limited White Noise/1 -> Sum1/1
  Integrator1/1 -> Sum2/2, Sum3/1
  Band-Limited White Noise1/1 -> Sum2/1
  " "/1 -> Sum3/2
  Sum3/1 -> Scope3/1, direction/1
  Gain1/1 -> Integrator1/1
  Sum2/1 -> Gain1/1
  Gain/1 -> Integrator/1
  Sum1/1 -> Gain/1
  Constant8/1 -> Gust/3(L)
  Gust/1(gust) -> Saturation/1
  Saturation/1 -> Sum/3, Scope/1
  Constant9/1 -> Gust/4(kappa2)
  Constant/1 -> Gust/2(u10)
  time/1 -> Gust/1(time)

== system part2_MAIN_2019_for_ayon_because_he_cant_update_his_matlab/Simulation 4/Current (North - East)/Subsystem ==
  Mux1 : Mux  Inputs=3
  Scope : Scope
  Step1 : Step  Time=0  After=0  SampleTime=0
  Step2 : Step  Time=0  After=-0.2  SampleTime=0
  Step3 : Step  Time=0  After=0  SampleTime=0
  Out1 : Outport
  wires:
  Mux1/1 -> Scope/1, Out1/1
  Step1/1 -> Mux1/1
  Step2/1 -> Mux1/2
  Step3/1 -> Mux1/3

== system part2_MAIN_2019_for_ayon_because_he_cant_update_his_matlab/Simulation 4/Current (North - East)/Subsystem1 ==
  Add : Sum  Inputs=+++
  Cos : Trigonometry  Operator=cos
  Gain : Gain  Gain=pi/180
  Matrix Multiply : Product
  Matrix Multiply1 : Product
  Mux : Mux  Inputs=3
  Ramp : simulink/Sources/Ramp  slope=0.45  start=2  InitialOutput=0
  Ramp1 : simulink/Sources/Ramp  slope=-0.45  start=202  InitialOutput=0
  Scope : Scope  NumInputPorts=3
  Sin : Trigonometry
  Step : Step  Time=2  After=0.5  SampleTime=0
  Step1 : Step  Time=2  Before=180  After=180  SampleTime=0
  Step2 : Step  Time=0  After=0  SampleTime=0
  Out1 : Outport
  wires:
  Step1/1 -> Add/1
  Ramp/1 -> Add/2
  Ramp1/1 -> Add/3
  Step/1 -> Matrix Multiply1/1, Matrix Multiply/1
  Sin/1 -> Matrix Multiply1/2, Scope/1
  Cos/1 -> Matrix Multiply/2, Scope/2
  Matrix Multiply/1 -> Mux/1
  Matrix Multiply1/1 -> Mux/2
  Step2/1 -> Mux/3
  Mux/1 -> Scope/3, Out1/1
  Add/1 -> Gain/1
  Gain/1 -> Sin/1, Cos/1

== system part2_MAIN_2019_for_ayon_because_he_cant_update_his_matlab/Simulation 4/Current (North - East)/Subsystem2 ==
  Mux : Mux  Inputs=3
  Step : Step  Time=0  After=0  SampleTime=0
  Out1 : Outport
  wires:
  Mux/1 -> Out1/1
  Step/1 -> Mux/3, Mux/2, Mux/1

== system part2_MAIN_2019_for_ayon_because_he_cant_update_his_matlab/Simulation 4/Observer/EKF ==
  note: selector
  y : Inport
  U : Inport  Port=2
  Constant : Constant  Value=M
  Constant1 : Constant  Value=D
  Constant10 : Constant  Value=Q
  Constant11 : Constant  Value=dt
  Constant12 : Constant  Value=inv_Tb
  Constant13 : Constant  Value=TAU
  Constant2 : Constant  Value=inv_M
  Constant3 : Constant  Value=Tb
  Constant4 : Constant  Value=Aw
  Constant5 : Constant  Value=Cw
  Constant6 : Constant  Value=B
  Constant7 : Constant  Value=H
  Constant8 : Constant  Value=E
  Constant9 : Constant  Value=R
  MATLAB Function : MATLAB Function  TreatAsAtomicUnit=on
  MATLAB Function1 : MATLAB Function  TreatAsAtomicUnit=on
  Memory : Memory  InitialCondition=zeros(15,1)
  Memory1 : Memory  InitialCondition=eye(15,15)
  Scope : Scope
  Scope2 : Scope
  Subsystem : Subsystem  Commented=on
  Subsystem1 : Subsystem  Commented=on
  Terminator : Terminator
  eta_hat : Outport
  nu_hat : Outport  Port=2
  wires:
  U/1 -> MATLAB Function/2(U)
  MATLAB Function1/1(eta_hat) -> eta_hat/1
  MATLAB Function/3(states_hat) -> MATLAB Function1/1(states_vector)
  MATLAB Function/4(error) -> Scope2/1
  y/1 -> MATLAB Function/1(y)
  MATLAB Function1/2(nu_hat) -> nu_hat/1
  MATLAB Function/2(states_update) -> Memory/1
  Constant/1 -> MATLAB Function/5(M)
  Constant1/1 -> MATLAB Function/6(D)
  Constant2/1 -> MATLAB Function/7(inv_M)
  Constant4/1 -> MATLAB Function/8(Aw)
  Constant3/1 -> MATLAB Function/9(Tb)
  Constant5/1 -> MATLAB Function/10(Cw)
  Constant8/1 -> MATLAB Function/11(E)
  Constant6/1 -> MATLAB Function/12(B)
  Constant7/1 -> MATLAB Function/13(H)
  Constant9/1 -> MATLAB Function/14(R)
  Constant10/1 -> MATLAB Function/15(Q)
  Constant11/1 -> MATLAB Function/16(dt)
  Constant12/1 -> MATLAB Function/17(inv_Tb)
  Constant13/1 -> MATLAB Function/18(TAU)
  Memory/1 -> MATLAB Function/4(states)
  MATLAB Function/1(P_update) -> Memory1/1, Scope/1
  Memory1/1 -> MATLAB Function/3(P)
  MATLAB Function/5(K) -> Terminator/1

== system part2_MAIN_2019_for_ayon_because_he_cant_update_his_matlab/Simulation 4/Observer/Passive Non-Linear ==
  note: eta_observer
  note: nu_observer
  note: Bias Estimator
  note: Wave Estimator: 1st order wave-induced motion
  y : Inport
  tau_est : Inport  Port=2
  Add : Sum
  Add1 : Sum  Inputs=++-
  Aw : Gain  Gain=WaveModel.A_w  Multiplication=Matrix(K*u)
  Cw : Gain  Gain=WaveModel.C_w  Multiplication=Matrix(K*u)
  Damping : Gain  Gain=Damping  Multiplication=Matrix(K*u)
  Integrator{,1..3} (4 alike) : Integrator
  K1 : Gain  Gain=npf.K_1  Multiplication=Matrix(K*u)
  K2 : Gain  Gain=npf.K_2  Multiplication=Matrix(K*u)
  K3 : Gain  Gain=npf.K_3  Multiplication=Matrix(K*u)
  K4 : Gain  Gain=npf.K_4  Multiplication=Matrix(K*u)
  M_inv : Gain  Gain=inv(ModelParams.Mass)  Multiplication=Matrix(K*u)
  Matrix Multiply : Product  Multiplication=Matrix(*)
  Matrix Multiply1 : Product  Multiplication=Matrix(*)
  Matrix Multiply2 : Product  Multiplication=Matrix(*)
  R_psi : MATLAB Function  TreatAsAtomicUnit=on
  R_psi_T : MATLAB Function  TreatAsAtomicUnit=on
  Subsystem : Subsystem
  Sum : Sum  Inputs=|++
  Sum1 : Sum  Inputs=|+-
  Sum2 : Sum  Inputs=|++
  Sum3 : Sum  Inputs=|++
  Sum4 : Sum  Inputs=|+-
  inv(Tb) : Gain  Gain=inv(Param.Tb)  Multiplication=Matrix(K*u)
  eta_hat : Outport
  nu_hat : Outport  Port=2
  wires:
  Matrix Multiply/1 -> Sum/1
  Matrix Multiply1/1 -> Add/2
  Matrix Multiply2/1 -> Add1/1  "R'b_hat"
  R_psi_T/1(y) -> Matrix Multiply/1, Matrix Multiply2/2
  Add1/1 -> M_inv/1
  Damping/1 -> Add1/3
  R_psi/1(y) -> Matrix Multiply1/1
  Sum/1 -> Add1/2  "R'k4y + tau"
  Add/1 -> Integrator3/1  "eta_hat_dot"
  inv(Tb)/1 -> Sum1/2
  y/1 -> Subsystem/1(y), Sum4/1  "y"
  Aw/1 -> Sum2/2
  K3/1 -> Sum1/1
  Cw/1 -> Sum3/1
  Integrator1/1 -> Cw/1, Aw/1  "zeta_hat"
  Sum1/1 -> Integrator2/1  "b_hat_dot"
  Integrator/1 -> nu_hat/1, Damping/1, Matrix Multiply1/2  "nu_hat"
  Sum4/1 -> K1/1, K2/1, K3/1, K4/1  "y_obs"
  Sum3/1 -> Sum4/2  "y_hat"
  Integrator3/1 -> eta_hat/1, Sum3/2  "eta_hat"
  Sum2/1 -> Integrator1/1
  K2/1 -> Add/1
  K4/1 -> Matrix Multiply/2
  M_inv/1 -> Integrator/1  "nu_hat_dot"
  Integrator2/1 -> inv(Tb)/1, Matrix Multiply2/1  "b_hat"
  tau_est/1 -> Sum/2
  K1/1 -> Sum2/1
  Subsystem/1(Out1) -> R_psi/1(u), R_psi_T/1(u)

== system part2_MAIN_2019_for_ayon_because_he_cant_update_his_matlab/Simulation 4/Observer/Subsystem ==
  In1 : Inport
  Demux : Demux  Outputs=6
  Mux : Mux  Inputs=3
  Terminator : Terminator
  Terminator1 : Terminator
  Terminator2 : Terminator
  Out1 : Outport
  wires:
  Mux/1 -> Out1/1
  Demux/6 -> Mux/3
  Demux/5 -> Terminator2/1
  Demux/2 -> Mux/2
  Demux/1 -> Mux/1
  Demux/3 -> Terminator/1
  In1/1 -> Demux/1
  Demux/4 -> Terminator1/1

== system part2_MAIN_2019_for_ayon_because_he_cant_update_his_matlab/Simulation 4/Reference Model/Simulation Selector ==
  Simulation 4 : Subsystem
  Out1 : Outport
  wires:
  Simulation 4/1(Out1) -> Out1/1

== system part2_MAIN_2019_for_ayon_because_he_cant_update_his_matlab/Simulation 4/Thrust Allocation/Unwrap ==
  alpha : Inport
  Demux : Demux  Outputs=5
  Mux : Mux  Inputs=5
  Unwrap : dspsigops/Unwrap  tol=pi  InputProcessing=Columns as channels (frame based)  running=off
  Unwrap1 : dspsigops/Unwrap  tol=pi  InputProcessing=Columns as channels (frame based)  running=off
  Unwrap2 : dspsigops/Unwrap  tol=pi  InputProcessing=Columns as channels (frame based)  running=off
  alpha [rad] : Outport
  wires:
  alpha/1 -> Demux/1
  Mux/1 -> alpha [rad]/1
  Demux/1 -> Mux/1
  Demux/4 -> Unwrap2/1
  Unwrap2/1 -> Mux/4
  Demux/5 -> Unwrap/1
  Unwrap/1 -> Mux/5
  Demux/3 -> Mux/3
  Demux/2 -> Unwrap1/1
  Unwrap1/1 -> Mux/2

== system part2_MAIN_2019_for_ayon_because_he_cant_update_his_matlab/Simulation 4/Thrust Allocation/Unwrap1 ==
  alpha : Inport
  Demux : Demux  Outputs=5
  Mux : Mux  Inputs=5
  Unwrap : dspsigops/Unwrap  tol=pi  InputProcessing=Columns as channels (frame based)  running=off
  Unwrap1 : dspsigops/Unwrap  tol=pi  InputProcessing=Columns as channels (frame based)  running=off
  Unwrap2 : dspsigops/Unwrap  tol=pi  InputProcessing=Columns as channels (frame based)  running=off
  alpha [rad] : Outport
  wires:
  Unwrap1/1 -> Mux/2
  Demux/2 -> Unwrap1/1
  Demux/3 -> Mux/3
  Unwrap/1 -> Mux/5
  Demux/5 -> Unwrap/1
  Unwrap2/1 -> Mux/4
  Demux/4 -> Unwrap2/1
  Demux/1 -> Mux/1
  Mux/1 -> alpha [rad]/1
  alpha/1 -> Demux/1

== system part2_MAIN_2019_for_ayon_because_he_cant_update_his_matlab/Simulation 4/Wind/V_w1 ==
  " " : Constant  Value=mean_wind_direction
  Band-Limited White Noise : simulink/Sources/Band-Limited White Noise  Cov=np_slow_varying  Ts=0.1  seed=[23341]
  Band-Limited White Noise1 : simulink/Sources/Band-Limited White Noise  Cov=np_direction  Ts=0.1  seed=[23341]
  Constant : Constant  Value=u10
  Constant1 : Constant  Value=kappa
  Constant2 : Constant  Value=height
  Constant3 : Constant  Value=u10
  Constant8 : Constant  Value=L
  Constant9 : Constant  Value=kappa2
  Gain : Gain  Gain=1/slow_varying_time_constant
  Gain1 : Gain  Gain=1/direction_time_constant
  Gust : MATLAB Function  TreatAsAtomicUnit=on
  Integrator : Integrator  LimitOutput=on  UpperSaturationLimit=slow_varying_limit  LowerSaturationLimit=-slow_varying_limit
  Integrator1 : Integrator  LimitOutput=on  UpperSaturationLimit=direction_limit  LowerSaturationLimit=-direction_limit
  Mean wind component : MATLAB Function  TreatAsAtomicUnit=on
  Saturation : Saturate  UpperLimit=gust_limit  LowerLimit=-10
  Scope{,1..3} (4 alike) : Scope
  Sum : Sum  Inputs=+|+|+
  Sum1 : Sum  Inputs=|+-
  Sum2 : Sum  Inputs=|+-
  Sum3 : Sum  Inputs=|++
  time : Clock
  wind : Outport
  direction : Outport  Port=2
  wires:
  Constant3/1 -> Mean wind component/1(u10)
  Constant1/1 -> Mean wind component/2(kappa)
  Constant2/1 -> Mean wind component/3(height)
  Mean wind component/1(mean_wind) -> Scope2/1, Sum/2
  Sum/1 -> wind/1
  Integrator/1 -> Scope1/1, Sum/1, Sum1/2
  Band-Limited White Noise/1 -> Sum1/1
  Integrator1/1 -> Sum2/2, Sum3/1
  Band-Limited White Noise1/1 -> Sum2/1
  " "/1 -> Sum3/2
  Sum3/1 -> Scope3/1, direction/1
  Gain1/1 -> Integrator1/1
  Sum2/1 -> Gain1/1
  Gain/1 -> Integrator/1
  Sum1/1 -> Gain/1
  Constant8/1 -> Gust/3(L)
  Gust/1(gust) -> Saturation/1
  Saturation/1 -> Sum/3, Scope/1
  Constant9/1 -> Gust/4(kappa2)
  Constant/1 -> Gust/2(u10)
  time/1 -> Gust/1(time)

== system part2_MAIN_2019_for_ayon_because_he_cant_update_his_matlab/Simulation 5/Current (North - East)/Subsystem ==
  Mux1 : Mux  Inputs=3
  Scope : Scope
  Step1 : Step  Time=0  After=0  SampleTime=0
  Step2 : Step  Time=0  After=-0.2  SampleTime=0
  Step3 : Step  Time=0  After=0  SampleTime=0
  Out1 : Outport
  wires:
  Mux1/1 -> Scope/1, Out1/1
  Step1/1 -> Mux1/1
  Step2/1 -> Mux1/2
  Step3/1 -> Mux1/3

== system part2_MAIN_2019_for_ayon_because_he_cant_update_his_matlab/Simulation 5/Current (North - East)/Subsystem1 ==
  Add : Sum  Inputs=+++
  Cos : Trigonometry  Operator=cos
  Gain : Gain  Gain=pi/180
  Matrix Multiply : Product
  Matrix Multiply1 : Product
  Mux : Mux  Inputs=3
  Ramp : simulink/Sources/Ramp  slope=0.45  start=2  InitialOutput=0
  Ramp1 : simulink/Sources/Ramp  slope=-0.45  start=202  InitialOutput=0
  Scope : Scope  NumInputPorts=3
  Sin : Trigonometry
  Step : Step  Time=2  After=0.5  SampleTime=0
  Step1 : Step  Time=2  Before=180  After=180  SampleTime=0
  Step2 : Step  Time=0  After=0  SampleTime=0
  Out1 : Outport
  wires:
  Step1/1 -> Add/1
  Ramp/1 -> Add/2
  Ramp1/1 -> Add/3
  Step/1 -> Matrix Multiply1/1, Matrix Multiply/1
  Sin/1 -> Matrix Multiply1/2, Scope/1
  Cos/1 -> Matrix Multiply/2, Scope/2
  Matrix Multiply/1 -> Mux/1
  Matrix Multiply1/1 -> Mux/2
  Step2/1 -> Mux/3
  Mux/1 -> Scope/3, Out1/1
  Add/1 -> Gain/1
  Gain/1 -> Sin/1, Cos/1

== system part2_MAIN_2019_for_ayon_because_he_cant_update_his_matlab/Simulation 5/Current (North - East)/Subsystem2 ==
  Mux : Mux  Inputs=3
  Step : Step  Time=0  After=0  SampleTime=0
  Out1 : Outport
  wires:
  Mux/1 -> Out1/1
  Step/1 -> Mux/3, Mux/2, Mux/1

== system part2_MAIN_2019_for_ayon_because_he_cant_update_his_matlab/Simulation 5/Observer/EKF ==
  note: selector
  y : Inport
  U : Inport  Port=2
  Constant : Constant  Value=M
  Constant1 : Constant  Value=D
  Constant10 : Constant  Value=Q
  Constant11 : Constant  Value=dt
  Constant12 : Constant  Value=inv_Tb
  Constant13 : Constant  Value=TAU
  Constant2 : Constant  Value=inv_M
  Constant3 : Constant  Value=Tb
  Constant4 : Constant  Value=Aw
  Constant5 : Constant  Value=Cw
  Constant6 : Constant  Value=B
  Constant7 : Constant  Value=H
  Constant8 : Constant  Value=E
  Constant9 : Constant  Value=R
  MATLAB Function : MATLAB Function  TreatAsAtomicUnit=on
  MATLAB Function1 : MATLAB Function  TreatAsAtomicUnit=on
  Memory : Memory  InitialCondition=zeros(15,1)
  Memory1 : Memory  InitialCondition=eye(15,15)
  Scope : Scope
  Scope2 : Scope
  Subsystem : Subsystem  Commented=on
  Subsystem1 : Subsystem  Commented=on
  Terminator : Terminator
  eta_hat : Outport
  nu_hat : Outport  Port=2
  wires:
  U/1 -> MATLAB Function/2(U)
  MATLAB Function1/1(eta_hat) -> eta_hat/1
  MATLAB Function/3(states_hat) -> MATLAB Function1/1(states_vector)
  MATLAB Function/4(error) -> Scope2/1
  y/1 -> MATLAB Function/1(y)
  MATLAB Function1/2(nu_hat) -> nu_hat/1
  MATLAB Function/2(states_update) -> Memory/1
  Constant/1 -> MATLAB Function/5(M)
  Constant1/1 -> MATLAB Function/6(D)
  Constant2/1 -> MATLAB Function/7(inv_M)
  Constant4/1 -> MATLAB Function/8(Aw)
  Constant3/1 -> MATLAB Function/9(Tb)
  Constant5/1 -> MATLAB Function/10(Cw)
  Constant8/1 -> MATLAB Function/11(E)
  Constant6/1 -> MATLAB Function/12(B)
  Constant7/1 -> MATLAB Function/13(H)
  Constant9/1 -> MATLAB Function/14(R)
  Constant10/1 -> MATLAB Function/15(Q)
  Constant11/1 -> MATLAB Function/16(dt)
  Constant12/1 -> MATLAB Function/17(inv_Tb)
  Constant13/1 -> MATLAB Function/18(TAU)
  Memory/1 -> MATLAB Function/4(states)
  MATLAB Function/1(P_update) -> Memory1/1, Scope/1
  Memory1/1 -> MATLAB Function/3(P)
  MATLAB Function/5(K) -> Terminator/1
